simulink model "three_phase_WPT"  (R2023a)
settings: Solver=FixedStepDiscrete  StartTime=0.0  StopTime=Tfinal  FixedStep=SampleTime  RelTol=1e-3
InitFcn:
  | param
values from neighbouring files (symbols this model uses):
  C_DCA = 150e-6    (= 0.00015)    [param.m]
  C_DCB = 150e-6    (= 0.00015)    [param.m]
  C_DCC = 150e-6    (= 0.00015)    [param.m]
  f_motor = 1000    [param.m]
  LSource = 1e-6    (= 1e-06)    [param.m]
  ma = 0.9    [param.m]
  ModuleAPhase = 0    [param.m]
  ModuleBPhase = 0    [param.m]
  ModuleCPhase = 0    [param.m]
  RSource = 0.01    [param.m]
  SampleTime = 1e-8    (= 1e-08)    [param.m]
  VDC = 1070    [param.m]
undefined symbols (not defined in the file or in its folder): C_DC, Cds, Cgd, Cgs, ESLA, ESLB, ESRA, ESRB, ESRC, LA_mid_parasitic, LA_parasitic, LAB_parasitic, LB_mid_parasitic, LB_parasitic, LBC_parasitic, LC_mid_parasitic, LC_parasitic, Lg, RA_mid_parasitic, RA_parasitic, RAB_parasitic, RB_mid_parasitic, RBC_parasitic, RC_mid_parasitic, rds, Rg
libraries: spsSeriesRLCBranchLib x26, spsCurrentMeasurementLib x10, spsVoltageMeasurementLib x7, spsMosfetLib x6, simulink x6, spsTriangleGeneratorLib x3, spsDCVoltageSourceLib x1, spsControlledCurrentSourceLib x1, spsControlledVoltageSourceLib x1, spspowerguiLib x1
settings Model: Creator=enes_  LastModifiedBy=enesa
settings SolverCC: AlgebraicLoopSolver=TrustRegion
settings DataIOCC: ReturnWorkspaceOutputs=off
settings DebuggingCC: UnconnectedInputMsg=warning  UnconnectedOutputMsg=warning  UnconnectedLineMsg=warning  ArithmeticOperatorsInVariantConditions=warning
settings ModelReferenceCC: EnableRefExpFcnMdlSchedulingChecks=on
settings SFSimCC: SimUseLocalCustomCode=off  CustomCodeUndefinedFunction=UseInterfaceOnly
settings RTWCC: RTWUseLocalCustomCode=off  DLArmComputeVersion=19.05

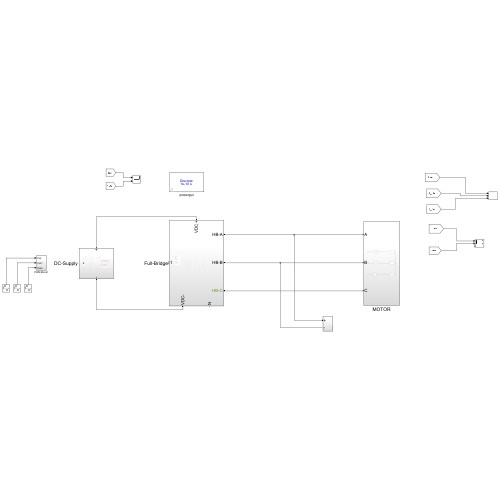
[thumbnail: Simulink's stored preview of the top-level diagram]
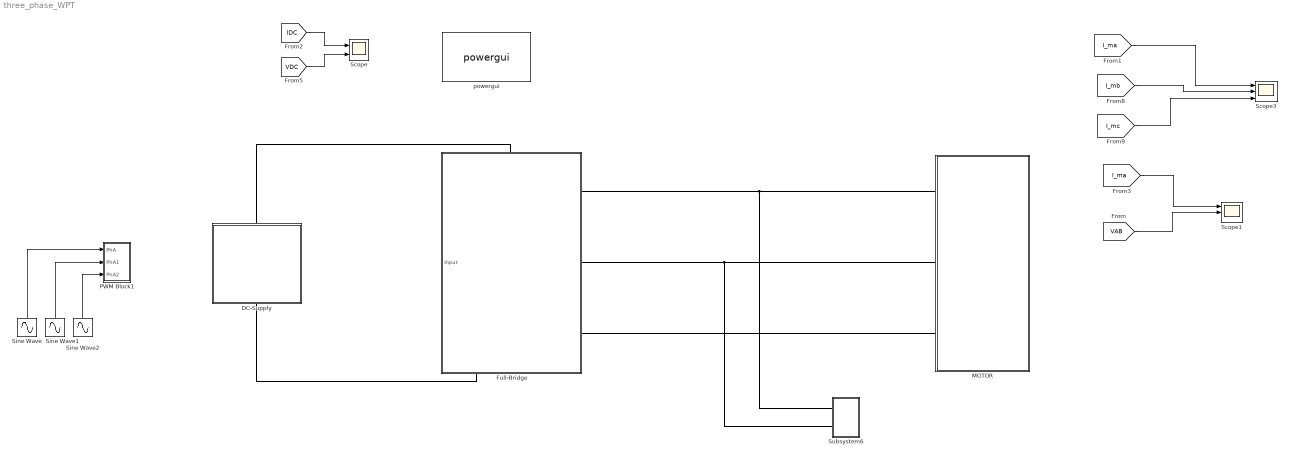
== system three_phase_WPT ==
  DC-Supply : Subsystem
  Full-Bridge : Subsystem
      settings: PortSchema="{\"entries\":[{\"content\":{\"sides\":[{\"content\":{\"connectorIds\":[\"In1\"]},\"type\":\"ConnectorPlacement.EquallySpacedRectSide\",\"uuid\":\"92c2640b-bb56-47f8-9c41-2323b38839f8\"},{\"content\":{\"connectorIds\":[\"RConn1\",\"RConn2\",\"RConn3\"],\"side\":\"RIGHT\"},\"type\":\"ConnectorPlacement.EquallySpacedRectSide\",\"uuid\":\"0b5c90a1-e2e1-4478-84c9-834496a6568e\"},{\"content\":{\"connectorIds\":[\"LConn1\"],\"side\":\"TOP\"},\"type\":\"ConnectorPlacement.EquallySpacedRectSide\",\"uuid\":\"1c803fb0-9096-4a7d-b495-aabd35d72306\"},{\"content\":{\"connectorIds\":[\"RConn4\",\"RConn5\"],\"side\":\"BOTTOM\"},\"type\":\"ConnectorPlacement.EquallySpacedRectSide\",\"uuid\":\"5a2d766c-8c3f-4943-ab0f-0e1988e2f8d8\"},{\"content\":{\"side\":\"HIDDEN\"},\"type\":\"ConnectorPlacement.EquallySpacedRectSide\",\"uuid\":\"8868c32c-a67f-4887-a91d-dc24242eaee2\"}]},\"type\":\"ConnectorPlacement.EquallySpacedConnector\",\"uuid\":\"a3546067-6216-40b0-bae0-9d71271c5112\"}],\"packageUris\":[\"http://schema.mathworks.com/mf0/Connector/R2020b\"],\"version\":\"1.0\"}"
  MOTOR : Subsystem
      settings: PortSchema="{\"entries\":[{\"content\":{\"sides\":[{\"content\":{\"connectorIds\":[]},\"type\":\"ConnectorPlacement.EquallySpacedRectSide\",\"uuid\":\"27af0988-5d70-46f2-9f63-66e4679735d7\"},{\"content\":{\"connectorIds\":[],\"side\":\"RIGHT\"},\"type\":\"ConnectorPlacement.EquallySpacedRectSide\",\"uuid\":\"9d673fb6-38db-4110-ad66-771dcf318fba\"},{\"content\":{\"connectorIds\":[\"LConn1\",\"LConn2\",\"LConn3\"],\"side\":\"TOP\"},\"type\":\"ConnectorPlacement.EquallySpacedRectSide\",\"uuid\":\"44eb7bd4-c702-4f50-84c2-cb9d75020b5b\"},{\"content\":{\"connectorIds\":[],\"side\":\"HIDDEN\"},\"type\":\"ConnectorPlacement.EquallySpacedRectSide\",\"uuid\":\"ba714e9b-5efc-4dbb-add8-803f06cf9de0\"}]},\"type\":\"ConnectorPlacement.EquallySpacedConnector\",\"uuid\":\"a2219d53-abb4-437b-a840-c37860cec52f\"}],\"packageUris\":[\"http://schema.mathworks.com/mf0/Connector/R2020b\"],\"version\":\"1.0\"}"
  PWM Block1 : Subsystem
  Scope : Scope  NumInputPorts=2
  Scope1 : Scope  NumInputPorts=3
  Scope3 : Scope  NumInputPorts=3
  Sine Wave : Sin  Amplitude=ma  Frequency=f_motor*2*pi  SampleTime=0
  Sine Wave1 : Sin  Amplitude=ma  Frequency=f_motor*2*pi  Phase=-2*pi/3  SampleTime=0
  Sine Wave2 : Sin  Amplitude=ma  Frequency=f_motor*2*pi  Phase=2*pi/3  SampleTime=0
  Subsystem6 : Subsystem
  powergui : spspowerguiLib/powergui  Priority=1  SimulationMode=Discrete  SampleTime=SampleTime  frequency=60  Iterations=50  frequencyindice=0  Pbase=100e6  ErrMax=1e-4  UnitsV=kV  UnitsW=MW  buscounter=0  FunctionMessages=off  echomessages=off  EnableUseOfTLC=off  CurrentSourceSwitches=off  DisableSnubberDevices=off  DisableRonSwitches=off  DisableVfSwitches=off  DisplayEquations=off  AutomaticDiscreteSolvers=off  SolverType=Tustin/Backward Euler (TBE)  Interpol=off  ExternalGateDelay=off  methode=off  Ts=100  x0status=blocks  SPID=on  SwTol=0  HookPort=off  NonlinearTolerance=1e-4  nMaxIteration=100  ContinueOnMaxIteration=off  RestoreLinks=warning  ResistiveCurrentMeasurement=off  Frange=[1e3:1e3:240e3]  Ylog=off  Xlog=on  ShowGrid=off  save=off  variable=ZData  structure=ScopeData2  ZoomFFT=off  StartTime=0.02  cycles=400  DisplayStyle=2  fundamental=80e3  FreqAxis=off  MaxFrequency=240e3  frequencyindicesteady=1  RmsSteady=1  display=off
  wires:
  [IDC] -> Scope/1
  [VDC] -> Scope/2
  [I_ma] -> Scope3/1
  [I_mb] -> Scope3/2
  [I_mc] -> Scope3/3
  Sine Wave2/1 -> PWM Block1/3(PhA2)
  Sine Wave1/1 -> PWM Block1/2(PhA1)
  Sine Wave/1 -> PWM Block1/1(PhA)
  [I_ma] -> Scope1/1
  [VAB] -> Scope1/2
  connections:
  DC-Supply/LConn1 -- Full-Bridge/LConn1
  DC-Supply/RConn1 -- Full-Bridge/RConn4
  Subsystem6/LConn1 -- Full-Bridge/RConn1 -- MOTOR/LConn1
  Full-Bridge/RConn2 -- Subsystem6/LConn2 -- MOTOR/LConn2
  Full-Bridge/RConn3 -- MOTOR/LConn3

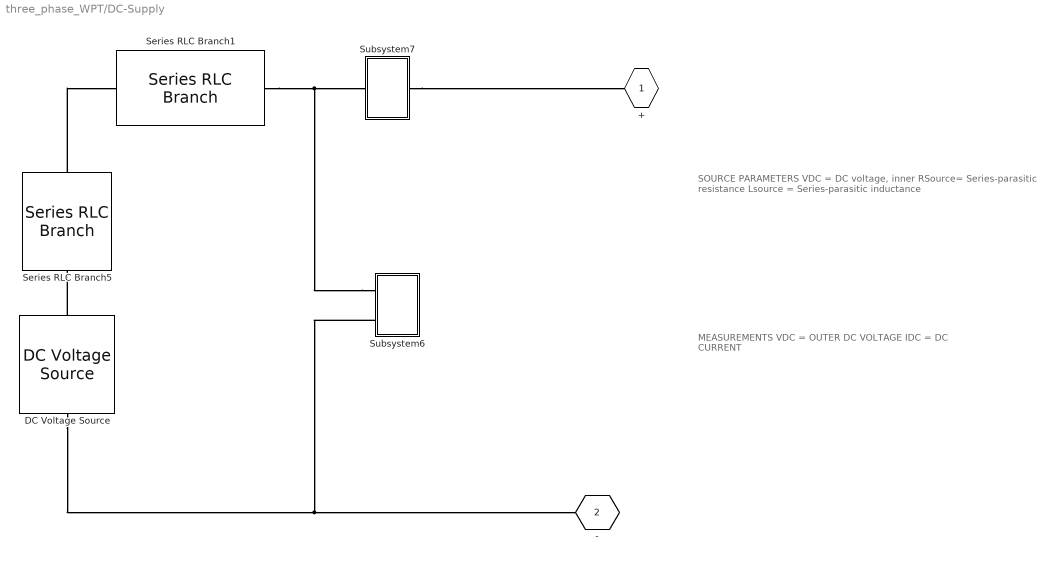
== system three_phase_WPT/DC-Supply ==
  note: SOURCE PARAMETERS
      | VDC = DC voltage, inner
      | RSource= Series-parasitic resistance
      | Lsource = Series-parasitic inductance
  note: MEASUREMENTS
      | VDC = OUTER DC VOLTAGE
      | IDC = DC CURRENT
  DC Voltage Source : spsDCVoltageSourceLib/DC Voltage Source  Amplitude=VDC  Measurements=None
  Series RLC Branch1 : spsSeriesRLCBranchLib/Series RLC Branch  LConnTagsString=__new0  RConnTagsString=__new0  BranchType=L  Resistance=LSource  Inductance=LSource  SetiL0=off  InitialCurrent=0  Capacitance=0.01  Setx0=off  InitialVoltage=0  Measurements=None
  Series RLC Branch5 : spsSeriesRLCBranchLib/Series RLC Branch  LConnTagsString=__new0  RConnTagsString=__new0  BranchType=R  Resistance=RSource  Inductance=ESLA  SetiL0=off  InitialCurrent=0  Capacitance=0.01  Setx0=off  InitialVoltage=0  Measurements=None
  Subsystem6 : Subsystem
  Subsystem7 : Subsystem
  + : PMIOPort  Side=Left
  - : PMIOPort  Port=2  Side=Right
  connections:
  Series RLC Branch5/LConn1 -- Series RLC Branch1/RConn1
  DC Voltage Source/LConn1 -- Subsystem6/LConn2 -- -/RConn1
  Subsystem6/LConn1 -- Series RLC Branch1/LConn1 -- Subsystem7/RConn1
  DC Voltage Source/RConn1 -- Series RLC Branch5/RConn1
  Subsystem7/LConn1 -- +/RConn1

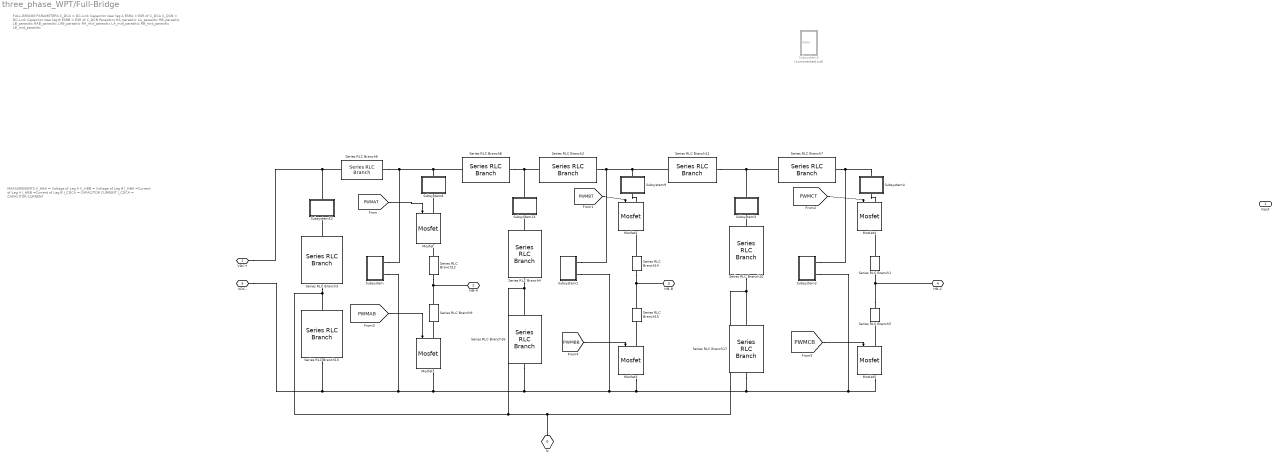
== system three_phase_WPT/Full-Bridge ==
  note: MEASUREMENTS
      | V_HBA = Voltage of Leg A
      | V_HBB = Voltage of Leg B
      | I_HBA =Current of Leg A
      | I_HBB =Current of Leg B
      | I_CDCA = CAPACITOR CURRENT
      | I_CDCA = CAPACITOR CURRENT
  note: FULL-BRIDGE PARAMETERS
      | C_DCA = DC-Link Capacitor near leg A
      | ESRA = ESR of C_DCA
      | C_DCB = DC-Link Capacitor near leg B
      | ESRB = ESR of C_DCB
      | Parasitics
      | RA_parasitic
      | LA_parasitic
      | RB_parasitic
      | LB_parasitic
      | RAB_parasitic
      | LAB_parasitic
      | RA_mid_parasitic
      | LA_mid_parasitic
      | RB_mid_parasitic
      | LB_mid_parasitic
  Input : Inport
  Mosfet{,1..5} (6 alike) : spsMosfetLib/Mosfet  Ron=0.1  Lon=0  Rd=0.01  Vfd=0  IC=0  Rs=1e5  Cs=inf  Measurements=on
  Series RLC Branch1 : spsSeriesRLCBranchLib/Series RLC Branch  LConnTagsString=__new0  RConnTagsString=__new0  BranchType=RL  Resistance=RC_mid_parasitic  Inductance=LC_mid_parasitic  SetiL0=off  InitialCurrent=0  Capacitance=C_DC  Setx0=off  InitialVoltage=0  Measurements=None
  Series RLC Branch10 : spsSeriesRLCBranchLib/Series RLC Branch  LConnTagsString=__new0  RConnTagsString=__new0  BranchType=RC  Resistance=ESRC  Inductance=ESLB  SetiL0=off  InitialCurrent=0  Capacitance=C_DCC  Setx0=off  InitialVoltage=0  Measurements=None
  Series RLC Branch11 : spsSeriesRLCBranchLib/Series RLC Branch  LConnTagsString=__new0  RConnTagsString=__new0  BranchType=RL  Resistance=RBC_parasitic  Inductance=LBC_parasitic  SetiL0=off  InitialCurrent=0  Capacitance=0.01  Setx0=off  InitialVoltage=0  Measurements=None
  Series RLC Branch12 : spsSeriesRLCBranchLib/Series RLC Branch  LConnTagsString=__new0  RConnTagsString=__new0  BranchType=RL  Resistance=RA_mid_parasitic  Inductance=LA_mid_parasitic  SetiL0=off  InitialCurrent=0  Capacitance=C_DC  Setx0=off  InitialVoltage=0  Measurements=None
  Series RLC Branch13 : spsSeriesRLCBranchLib/Series RLC Branch  LConnTagsString=__new0  RConnTagsString=__new0  BranchType=RC  Resistance=ESRA  Inductance=ESLA  SetiL0=off  InitialCurrent=0  Capacitance=C_DCA  Setx0=off  InitialVoltage=0  Measurements=None
  Series RLC Branch14 : spsSeriesRLCBranchLib/Series RLC Branch  LConnTagsString=__new0  RConnTagsString=__new0  BranchType=RL  Resistance=RB_mid_parasitic  Inductance=LB_mid_parasitic  SetiL0=off  InitialCurrent=0  Capacitance=C_DC  Setx0=off  InitialVoltage=0  Measurements=None
  Series RLC Branch15 : spsSeriesRLCBranchLib/Series RLC Branch  LConnTagsString=__new0  RConnTagsString=__new0  BranchType=RL  Resistance=RB_mid_parasitic  Inductance=LB_mid_parasitic  SetiL0=off  InitialCurrent=0  Capacitance=C_DC  Setx0=off  InitialVoltage=0  Measurements=None
  Series RLC Branch16 : spsSeriesRLCBranchLib/Series RLC Branch  LConnTagsString=__new0  RConnTagsString=__new0  BranchType=RC  Resistance=ESRB  Inductance=ESLB  SetiL0=off  InitialCurrent=0  Capacitance=C_DCB  Setx0=off  InitialVoltage=0  Measurements=None
  Series RLC Branch17 : spsSeriesRLCBranchLib/Series RLC Branch  LConnTagsString=__new0  RConnTagsString=__new0  BranchType=RC  Resistance=ESRB  Inductance=ESLB  SetiL0=off  InitialCurrent=0  Capacitance=C_DCB  Setx0=off  InitialVoltage=0  Measurements=None
  Series RLC Branch2 : spsSeriesRLCBranchLib/Series RLC Branch  LConnTagsString=__new0  RConnTagsString=__new0  BranchType=RL  Resistance=LB_parasitic  Inductance=LB_parasitic  SetiL0=off  InitialCurrent=0  Capacitance=0.01  Setx0=off  InitialVoltage=0  Measurements=None
  Series RLC Branch3 : spsSeriesRLCBranchLib/Series RLC Branch  LConnTagsString=__new0  RConnTagsString=__new0  BranchType=RC  Resistance=ESRA  Inductance=ESLA  SetiL0=off  InitialCurrent=0  Capacitance=C_DCA  Setx0=off  InitialVoltage=0  Measurements=None
  Series RLC Branch4 : spsSeriesRLCBranchLib/Series RLC Branch  LConnTagsString=__new0  RConnTagsString=__new0  BranchType=RC  Resistance=ESRB  Inductance=ESLB  SetiL0=off  InitialCurrent=0  Capacitance=C_DCB  Setx0=off  InitialVoltage=0  Measurements=None
  Series RLC Branch5 : spsSeriesRLCBranchLib/Series RLC Branch  LConnTagsString=__new0  RConnTagsString=__new0  BranchType=RL  Resistance=RC_mid_parasitic  Inductance=LC_mid_parasitic  SetiL0=off  InitialCurrent=0  Capacitance=C_DC  Setx0=off  InitialVoltage=0  Measurements=None
  Series RLC Branch6 : spsSeriesRLCBranchLib/Series RLC Branch  LConnTagsString=__new0  RConnTagsString=__new0  BranchType=RL  Resistance=RA_parasitic  Inductance=LA_parasitic  SetiL0=off  InitialCurrent=0  Capacitance=0.01  Setx0=off  InitialVoltage=0  Measurements=None
  Series RLC Branch7 : spsSeriesRLCBranchLib/Series RLC Branch  LConnTagsString=__new0  RConnTagsString=__new0  BranchType=RL  Resistance=LC_parasitic  Inductance=LC_parasitic  SetiL0=off  InitialCurrent=0  Capacitance=0.01  Setx0=off  InitialVoltage=0  Measurements=None
  Series RLC Branch8 : spsSeriesRLCBranchLib/Series RLC Branch  LConnTagsString=__new0  RConnTagsString=__new0  BranchType=RL  Resistance=RAB_parasitic  Inductance=LAB_parasitic  SetiL0=off  InitialCurrent=0  Capacitance=0.01  Setx0=off  InitialVoltage=0  Measurements=None
  Series RLC Branch9 : spsSeriesRLCBranchLib/Series RLC Branch  LConnTagsString=__new0  RConnTagsString=__new0  BranchType=RL  Resistance=RA_mid_parasitic  Inductance=LA_mid_parasitic  SetiL0=off  InitialCurrent=0  Capacitance=C_DC  Setx0=off  InitialVoltage=0  Measurements=None
  Subsystem : Subsystem
  Subsystem1 : Subsystem
  Subsystem12 : Subsystem
  Subsystem13 : Subsystem
  Subsystem2 : Subsystem
  Subsystem3 : Subsystem
  Subsystem4 : Subsystem
  Subsystem5 : Subsystem  Commented=on
  Subsystem8 : Subsystem
  Subsystem9 : Subsystem
  VDC+ : PMIOPort  Side=Left
  HB-A : PMIOPort  Port=2  Side=Right
  HB-B : PMIOPort  Port=3  Side=Right
  HB-C : PMIOPort  Port=4  Side=Right
  VDC- : PMIOPort  Port=5  Side=Right
  N : PMIOPort  Port=6  Side=Right
  wires:
  [PWMAB] -> Mosfet1/1
  [PWMAT] -> Mosfet/1
  [PWMBB] -> Mosfet3/1
  [PWMBT] -> Mosfet2/1
  [PWMCT] -> Mosfet4/1
  [PWMCB] -> Mosfet5/1
  connections:
  Subsystem13/RConn1 -- Series RLC Branch8/LConn1 -- Series RLC Branch2/RConn1
  VDC+/RConn1 -- Subsystem12/RConn1 -- Series RLC Branch6/RConn1
  Mosfet1/LConn1 -- Series RLC Branch9/LConn1
  Series RLC Branch6/LConn1 -- Subsystem/LConn1 -- Subsystem8/RConn1 -- Series RLC Branch8/RConn1
  Mosfet3/LConn1 -- Series RLC Branch15/LConn1
  Subsystem9/LConn1 -- Mosfet2/LConn1
  Series RLC Branch4/LConn1 -- Subsystem13/LConn1
  Series RLC Branch3/LConn1 -- Subsystem12/LConn1
  Series RLC Branch14/RConn1 -- Mosfet2/RConn1
  Series RLC Branch2/LConn1 -- Subsystem1/LConn1 -- Series RLC Branch11/RConn1 -- Subsystem9/RConn1
  Series RLC Branch12/RConn1 -- Mosfet/RConn1
  Mosfet/LConn1 -- Subsystem8/LConn1
  HB-B/RConn1 -- Series RLC Branch14/LConn1 -- Series RLC Branch15/RConn1
  Series RLC Branch12/LConn1 -- HB-A/RConn1 -- Series RLC Branch9/RConn1
  Subsystem4/RConn1 -- Series RLC Branch7/LConn1 -- Subsystem2/LConn1
  Series RLC Branch5/RConn1 -- HB-C/RConn1 -- Series RLC Branch1/LConn1
  Series RLC Branch11/LConn1 -- Series RLC Branch7/RConn1 -- Subsystem3/RConn1
  Series RLC Branch1/RConn1 -- Mosfet4/RConn1
  Series RLC Branch10/LConn1 -- Subsystem3/LConn1
  Mosfet5/LConn1 -- Series RLC Branch5/LConn1
  Subsystem4/LConn1 -- Mosfet4/LConn1
  Series RLC Branch10/RConn1 -- Series RLC Branch16/LConn1 -- Series RLC Branch4/RConn1 -- Series RLC Branch13/LConn1 -- Series RLC Branch3/RConn1 -- N/RConn1 -- Series RLC Branch17/LConn1
  Series RLC Branch13/RConn1 -- Series RLC Branch16/RConn1 -- Series RLC Branch17/RConn1 -- Subsystem2/LConn2 -- Mosfet5/RConn1 -- Mosfet3/RConn1 -- Subsystem1/LConn2 -- Mosfet1/RConn1 -- Subsystem/LConn2 -- VDC-/RConn1

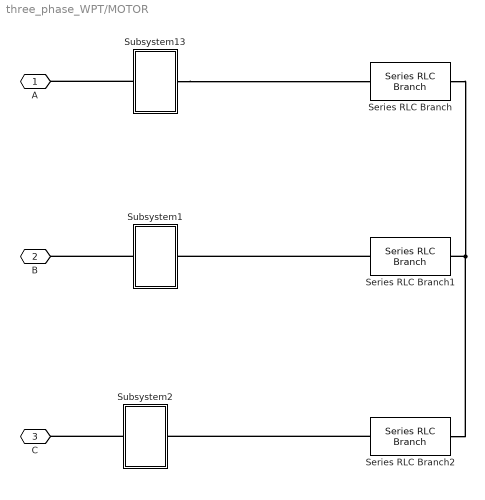
== system three_phase_WPT/MOTOR ==
  Series RLC Branch : spsSeriesRLCBranchLib/Series RLC Branch  LConnTagsString=__new0  RConnTagsString=__new0  BranchType=RL  Resistance=10  Inductance=4e-3  SetiL0=off  InitialCurrent=0  Capacitance=1e-6  Setx0=off  InitialVoltage=0  Measurements=None
  Series RLC Branch1 : spsSeriesRLCBranchLib/Series RLC Branch  LConnTagsString=__new0  RConnTagsString=__new0  BranchType=RL  Resistance=10  Inductance=4e-3  SetiL0=off  InitialCurrent=0  Capacitance=1e-6  Setx0=off  InitialVoltage=0  Measurements=None
  Series RLC Branch2 : spsSeriesRLCBranchLib/Series RLC Branch  LConnTagsString=__new0  RConnTagsString=__new0  BranchType=RL  Resistance=10  Inductance=4e-3  SetiL0=off  InitialCurrent=0  Capacitance=1e-6  Setx0=off  InitialVoltage=0  Measurements=None
  Subsystem1 : Subsystem
  Subsystem13 : Subsystem
  Subsystem2 : Subsystem
  A : PMIOPort  Side=Left
  B : PMIOPort  Port=2  Side=Left
  C : PMIOPort  Port=3  Side=Left
  connections:
  Subsystem13/LConn1 -- Series RLC Branch/LConn1
  Subsystem13/RConn1 -- A/RConn1
  Subsystem1/RConn1 -- B/RConn1
  Subsystem2/RConn1 -- C/RConn1
  Series RLC Branch1/LConn1 -- Subsystem1/LConn1
  Series RLC Branch2/LConn1 -- Subsystem2/LConn1
  Series RLC Branch/RConn1 -- Series RLC Branch2/RConn1 -- Series RLC Branch1/RConn1

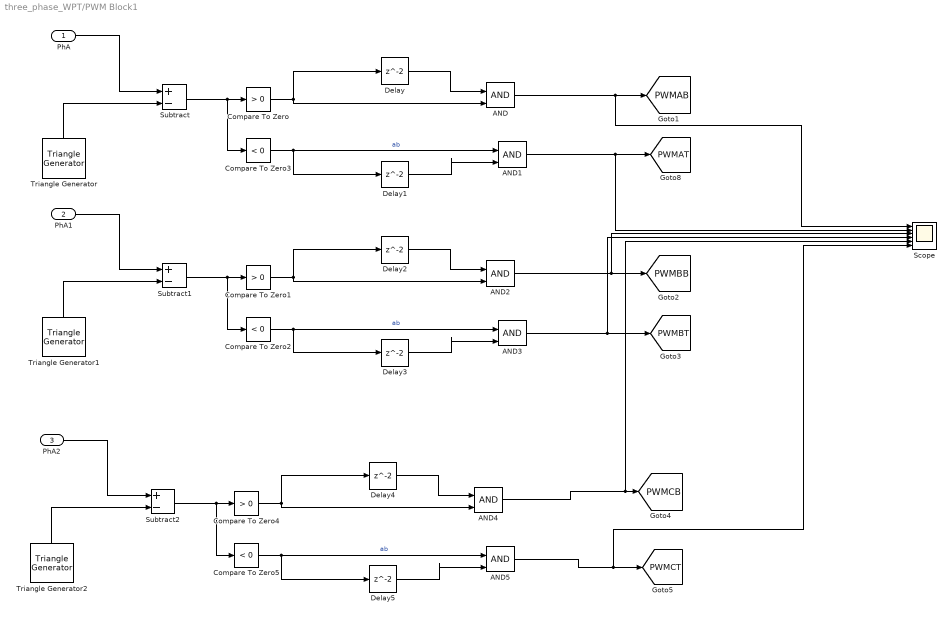
== system three_phase_WPT/PWM Block1 ==
  PhA : Inport
  PhA1 : Inport  Port=2
  PhA2 : Inport  Port=3
  AND{,1..5} (6 alike) : Logic  IconShape=distinctive  AllPortsSameDT=off  OutDataTypeStr=boolean
  Compare To Zero : simulink/Logic and Bit Operations/Compare To Zero  relop=>  OutDataTypeStr=boolean
  Compare To Zero1 : simulink/Logic and Bit Operations/Compare To Zero  relop=>  OutDataTypeStr=boolean
  Compare To Zero2 : simulink/Logic and Bit Operations/Compare To Zero  relop=<  OutDataTypeStr=boolean
  Compare To Zero3 : simulink/Logic and Bit Operations/Compare To Zero  relop=<  OutDataTypeStr=boolean
  Compare To Zero4 : simulink/Logic and Bit Operations/Compare To Zero  relop=>  OutDataTypeStr=boolean
  Compare To Zero5 : simulink/Logic and Bit Operations/Compare To Zero  relop=<  OutDataTypeStr=boolean
  Delay{,1..5} (6 alike) : Delay
  Scope : Scope  NumInputPorts=6
  Subtract : Sum  Inputs=+-
  Subtract1 : Sum  Inputs=+-
  Subtract2 : Sum  Inputs=+-
  Triangle Generator : spsTriangleGeneratorLib/Triangle Generator  Freq=fsw  Phase=ModuleAPhase  Ts=SampleTime
  Triangle Generator1 : spsTriangleGeneratorLib/Triangle Generator  Freq=fsw  Phase=ModuleBPhase  Ts=SampleTime
  Triangle Generator2 : spsTriangleGeneratorLib/Triangle Generator  Freq=fsw  Phase=ModuleCPhase  Ts=SampleTime
  tag scope: PWMAB=global, PWMAT=global, PWMBB=global, PWMBT=global, PWMCB=global, PWMCT=global
  wires:
  PhA/1 -> Subtract/1
  Triangle Generator/1 -> Subtract/2
  Subtract/1 -> Compare To Zero3/1, Compare To Zero/1
  Compare To Zero/1 -> Delay/1, AND/2
  Delay/1 -> AND/1
  Compare To Zero3/1 -> Delay1/1, AND1/1  "ab"
  Delay1/1 -> AND1/2
  AND2/1 -> Scope/3, [PWMBB]
  AND/1 -> Scope/1, [PWMAB]
  AND4/1 -> Scope/5, [PWMCB]
  Delay3/1 -> AND3/2
  Compare To Zero1/1 -> Delay2/1, AND2/2
  Delay2/1 -> AND2/1
  Compare To Zero2/1 -> Delay3/1, AND3/1  "ab"
  Subtract1/1 -> Compare To Zero2/1, Compare To Zero1/1
  Triangle Generator1/1 -> Subtract1/2
  PhA1/1 -> Subtract1/1
  Delay5/1 -> AND5/2
  Compare To Zero4/1 -> Delay4/1, AND4/2
  Delay4/1 -> AND4/1
  Compare To Zero5/1 -> Delay5/1, AND5/1  "ab"
  Subtract2/1 -> Compare To Zero5/1, Compare To Zero4/1
  Triangle Generator2/1 -> Subtract2/2
  PhA2/1 -> Subtract2/1
  AND1/1 -> Scope/2, [PWMAT]
  AND3/1 -> Scope/4, [PWMBT]
  AND5/1 -> Scope/6, [PWMCT]

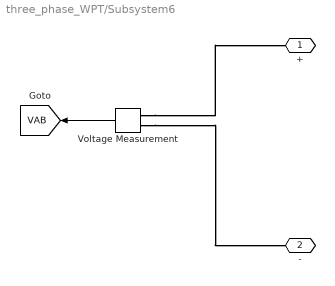
== system three_phase_WPT/Subsystem6 ==
  Voltage Measurement : spsVoltageMeasurementLib/Voltage Measurement  PhasorSimulation=off  OutputType=Complex  PSBequivalent=0
  + : PMIOPort  Side=Left
  - : PMIOPort  Port=2  Side=Left
  tag scope: VAB=global
  wires:
  Voltage Measurement/1 -> [VAB]
  connections:
  Voltage Measurement/LConn1 -- +/RConn1
  Voltage Measurement/LConn2 -- -/RConn1

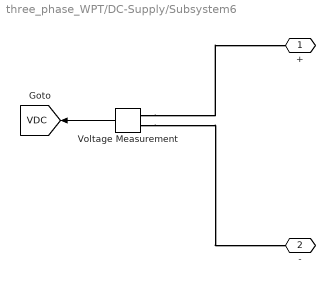
== system three_phase_WPT/DC-Supply/Subsystem6 ==
  Voltage Measurement : spsVoltageMeasurementLib/Voltage Measurement  PhasorSimulation=off  OutputType=Complex  PSBequivalent=0
  + : PMIOPort  Side=Left
  - : PMIOPort  Port=2  Side=Left
  tag scope: VDC=global
  wires:
  Voltage Measurement/1 -> [VDC]
  connections:
  Voltage Measurement/LConn1 -- +/RConn1
  Voltage Measurement/LConn2 -- -/RConn1

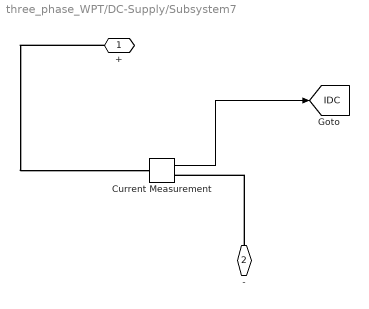
== system three_phase_WPT/DC-Supply/Subsystem7 ==
  Current Measurement : spsCurrentMeasurementLib/Current Measurement  PhasorSimulation=off  OutputType=Complex  PSBequivalent=0
  + : PMIOPort  Side=Right
  - : PMIOPort  Port=2  Side=Left
  tag scope: IDC=global
  wires:
  Current Measurement/1 -> [IDC]
  connections:
  +/RConn1 -- Current Measurement/LConn1
  -/RConn1 -- Current Measurement/RConn1

== system three_phase_WPT/Full-Bridge/Subsystem ==
  Voltage Measurement : spsVoltageMeasurementLib/Voltage Measurement  PhasorSimulation=off  OutputType=Complex  PSBequivalent=0
  + : PMIOPort  Side=Left
  - : PMIOPort  Port=2  Side=Left
  tag scope: V_HBA=global
  wires:
  Voltage Measurement/1 -> [V_HBA]
  connections:
  Voltage Measurement/LConn1 -- +/RConn1
  Voltage Measurement/LConn2 -- -/RConn1

== system three_phase_WPT/Full-Bridge/Subsystem1 ==
  Voltage Measurement : spsVoltageMeasurementLib/Voltage Measurement  PhasorSimulation=off  OutputType=Complex  PSBequivalent=0
  + : PMIOPort  Side=Left
  - : PMIOPort  Port=2  Side=Left
  tag scope: V_HBB=global
  wires:
  Voltage Measurement/1 -> [V_HBB]
  connections:
  Voltage Measurement/LConn1 -- +/RConn1
  Voltage Measurement/LConn2 -- -/RConn1

== system three_phase_WPT/Full-Bridge/Subsystem12 ==
  Current Measurement : spsCurrentMeasurementLib/Current Measurement  PhasorSimulation=off  OutputType=Complex  PSBequivalent=0
  + : PMIOPort  Side=Right
  - : PMIOPort  Port=2  Side=Left
  tag scope: IC_DCA=global
  wires:
  Current Measurement/1 -> [IC_DCA]
  connections:
  +/RConn1 -- Current Measurement/LConn1
  -/RConn1 -- Current Measurement/RConn1

== system three_phase_WPT/Full-Bridge/Subsystem13 ==
  Current Measurement : spsCurrentMeasurementLib/Current Measurement  PhasorSimulation=off  OutputType=Complex  PSBequivalent=0
  + : PMIOPort  Side=Right
  - : PMIOPort  Port=2  Side=Left
  tag scope: I_CDCB=global
  wires:
  Current Measurement/1 -> [I_CDCB]
  connections:
  +/RConn1 -- Current Measurement/LConn1
  -/RConn1 -- Current Measurement/RConn1

== system three_phase_WPT/Full-Bridge/Subsystem2 ==
  Voltage Measurement : spsVoltageMeasurementLib/Voltage Measurement  PhasorSimulation=off  OutputType=Complex  PSBequivalent=0
  + : PMIOPort  Side=Left
  - : PMIOPort  Port=2  Side=Left
  tag scope: V_HBC=global
  wires:
  Voltage Measurement/1 -> [V_HBC]
  connections:
  Voltage Measurement/LConn1 -- +/RConn1
  Voltage Measurement/LConn2 -- -/RConn1

== system three_phase_WPT/Full-Bridge/Subsystem3 ==
  Current Measurement : spsCurrentMeasurementLib/Current Measurement  PhasorSimulation=off  OutputType=Complex  PSBequivalent=0
  + : PMIOPort  Side=Right
  - : PMIOPort  Port=2  Side=Left
  tag scope: I_CDCC=global
  wires:
  Current Measurement/1 -> [I_CDCC]
  connections:
  +/RConn1 -- Current Measurement/LConn1
  -/RConn1 -- Current Measurement/RConn1

== system three_phase_WPT/Full-Bridge/Subsystem4 ==
  Current Measurement : spsCurrentMeasurementLib/Current Measurement  PhasorSimulation=off  OutputType=Complex  PSBequivalent=0
  + : PMIOPort  Side=Right
  - : PMIOPort  Port=2  Side=Left
  tag scope: I_HBC=global
  wires:
  Current Measurement/1 -> [I_HBC]
  connections:
  +/RConn1 -- Current Measurement/LConn1
  -/RConn1 -- Current Measurement/RConn1

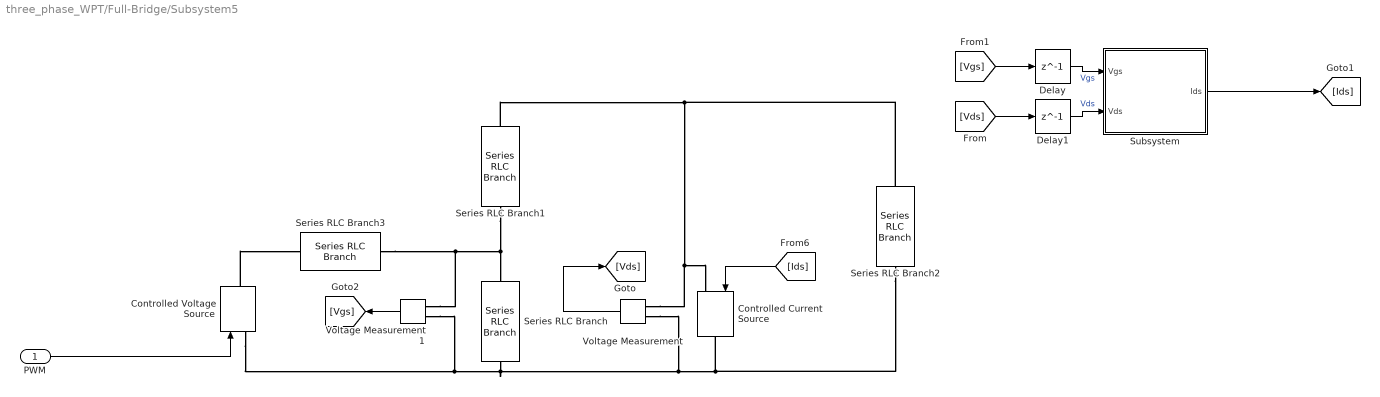
== system three_phase_WPT/Full-Bridge/Subsystem5 ==
  PWM : Inport
  Controlled Current Source : spsControlledCurrentSourceLib/Controlled Current Source  Initialize=on  Source_Type=AC  Amplitude=0  Phase=0  Frequency=0  Measurements=None
  Controlled Voltage Source : spsControlledVoltageSourceLib/Controlled Voltage Source  Initialize=on  Source_Type=AC  Amplitude=0  Phase=0  Frequency=0  Measurements=None
  Delay : Delay  DelayLength=1
  Delay1 : Delay  DelayLength=1
  Series RLC Branch : spsSeriesRLCBranchLib/Series RLC Branch  LConnTagsString=__new0  RConnTagsString=__new0  BranchType=C  Resistance=1  Inductance=1e-3  SetiL0=off  InitialCurrent=0  Capacitance=Cgs  Setx0=off  InitialVoltage=0  Measurements=None
  Series RLC Branch1 : spsSeriesRLCBranchLib/Series RLC Branch  LConnTagsString=__new0  RConnTagsString=__new0  BranchType=C  Resistance=1  Inductance=1e-3  SetiL0=off  InitialCurrent=0  Capacitance=Cgd  Setx0=off  InitialVoltage=0  Measurements=None
  Series RLC Branch2 : spsSeriesRLCBranchLib/Series RLC Branch  LConnTagsString=__new0  RConnTagsString=__new0  BranchType=C  Resistance=1  Inductance=1e-3  SetiL0=off  InitialCurrent=0  Capacitance=Cds  Setx0=off  InitialVoltage=0  Measurements=None
  Series RLC Branch3 : spsSeriesRLCBranchLib/Series RLC Branch  LConnTagsString=__new0  RConnTagsString=__new0  BranchType=RL  Resistance=Rg  Inductance=Lg  SetiL0=off  InitialCurrent=0  Capacitance=Cgs  Setx0=off  InitialVoltage=0  Measurements=None
  Subsystem : Subsystem
  Voltage Measurement : spsVoltageMeasurementLib/Voltage Measurement  PhasorSimulation=off  OutputType=Complex  PSBequivalent=0
  Voltage Measurement1 : spsVoltageMeasurementLib/Voltage Measurement  PhasorSimulation=off  OutputType=Complex  PSBequivalent=0
  wires:
  [Ids] -> Controlled Current Source/1
  Voltage Measurement/1 -> [Vds]
  PWM/1 -> Controlled Voltage Source/1
  Voltage Measurement1/1 -> [Vgs]
  [Vgs] -> Delay/1
  [Vds] -> Delay1/1
  Delay/1 -> Subsystem/1(Vgs)  "Vgs"
  Delay1/1 -> Subsystem/2(Vds)  "Vds"
  Subsystem/1(Ids) -> [Ids]
  connections:
  Series RLC Branch/RConn1 -- Controlled Voltage Source/LConn1 -- Voltage Measurement1/LConn2 -- Voltage Measurement/LConn2 -- Series RLC Branch2/RConn1 -- Controlled Current Source/RConn1
  Series RLC Branch1/LConn1 -- Series RLC Branch2/LConn1 -- Voltage Measurement/LConn1 -- Controlled Current Source/LConn1
  Series RLC Branch1/RConn1 -- Voltage Measurement1/LConn1 -- Series RLC Branch3/LConn1 -- Series RLC Branch/LConn1
  Controlled Voltage Source/RConn1 -- Series RLC Branch3/RConn1

== system three_phase_WPT/Full-Bridge/Subsystem8 ==
  Current Measurement : spsCurrentMeasurementLib/Current Measurement  PhasorSimulation=off  OutputType=Complex  PSBequivalent=0
  + : PMIOPort  Side=Right
  - : PMIOPort  Port=2  Side=Left
  tag scope: I_HBA=global
  wires:
  Current Measurement/1 -> [I_HBA]
  connections:
  +/RConn1 -- Current Measurement/LConn1
  -/RConn1 -- Current Measurement/RConn1

== system three_phase_WPT/Full-Bridge/Subsystem9 ==
  Current Measurement : spsCurrentMeasurementLib/Current Measurement  PhasorSimulation=off  OutputType=Complex  PSBequivalent=0
  + : PMIOPort  Side=Right
  - : PMIOPort  Port=2  Side=Left
  tag scope: I_HBB=global
  wires:
  Current Measurement/1 -> [I_HBB]
  connections:
  +/RConn1 -- Current Measurement/LConn1
  -/RConn1 -- Current Measurement/RConn1

== system three_phase_WPT/MOTOR/Subsystem1 ==
  Current Measurement : spsCurrentMeasurementLib/Current Measurement  PhasorSimulation=off  OutputType=Complex  PSBequivalent=0
  + : PMIOPort  Side=Right
  - : PMIOPort  Port=2  Side=Left
  tag scope: I_mb=global
  wires:
  Current Measurement/1 -> [I_mb]
  connections:
  +/RConn1 -- Current Measurement/LConn1
  -/RConn1 -- Current Measurement/RConn1

== system three_phase_WPT/MOTOR/Subsystem13 ==
  Current Measurement : spsCurrentMeasurementLib/Current Measurement  PhasorSimulation=off  OutputType=Complex  PSBequivalent=0
  + : PMIOPort  Side=Right
  - : PMIOPort  Port=2  Side=Left
  tag scope: I_ma=global
  wires:
  Current Measurement/1 -> [I_ma]
  connections:
  +/RConn1 -- Current Measurement/LConn1
  -/RConn1 -- Current Measurement/RConn1

== system three_phase_WPT/MOTOR/Subsystem2 ==
  Current Measurement : spsCurrentMeasurementLib/Current Measurement  PhasorSimulation=off  OutputType=Complex  PSBequivalent=0
  + : PMIOPort  Side=Right
  - : PMIOPort  Port=2  Side=Left
  tag scope: I_mc=global
  wires:
  Current Measurement/1 -> [I_mc]
  connections:
  +/RConn1 -- Current Measurement/LConn1
  -/RConn1 -- Current Measurement/RConn1

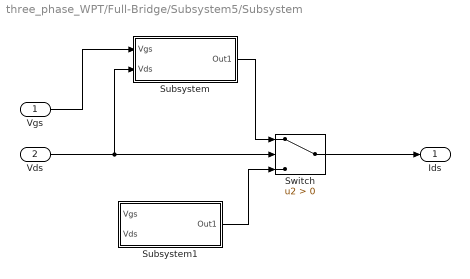
== system three_phase_WPT/Full-Bridge/Subsystem5/Subsystem ==
  Vgs : Inport
  Vds : Inport  Port=2
  Subsystem : Subsystem
  Subsystem1 : Subsystem
  Switch : Switch  Criteria=u2 > Threshold  SaturateOnIntegerOverflow=off  InputSameDT=off
  Ids : Outport
  wires:
  Switch/1 -> Ids/1
  Vds/1 -> Subsystem/2(Vds), Switch/2
  Vgs/1 -> Subsystem/1(Vgs)
  Subsystem/1(Out1) -> Switch/1
  Subsystem1/1(Out1) -> Switch/3

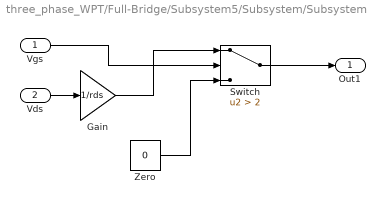
== system three_phase_WPT/Full-Bridge/Subsystem5/Subsystem/Subsystem ==
  Vgs : Inport
  Vds : Inport  Port=2
  Gain : Gain  Gain=1/rds
  Switch : Switch  Criteria=u2 > Threshold  Threshold=2  SaturateOnIntegerOverflow=off  InputSameDT=off
  Zero : Constant  Value=0  OutDataTypeStr=Inherit: Inherit via back propagation
  Out1 : Outport
  wires:
  Vgs/1 -> Switch/2
  Zero/1 -> Switch/3
  Switch/1 -> Out1/1
  Vds/1 -> Gain/1
  Gain/1 -> Switch/1

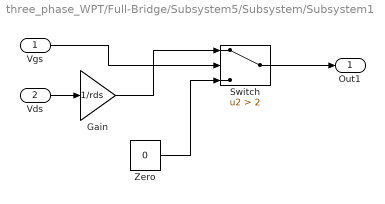
== system three_phase_WPT/Full-Bridge/Subsystem5/Subsystem/Subsystem1 ==
  Vgs : Inport
  Vds : Inport  Port=2
  Gain : Gain  Gain=1/rds
  Switch : Switch  Criteria=u2 > Threshold  Threshold=2  SaturateOnIntegerOverflow=off  InputSameDT=off
  Zero : Constant  Value=0  OutDataTypeStr=Inherit: Inherit via back propagation
  Out1 : Outport
  wires:
  Vgs/1 -> Switch/2
  Zero/1 -> Switch/3
  Switch/1 -> Out1/1
  Vds/1 -> Gain/1
  Gain/1 -> Switch/1
